simulink model "pam_demod"  (R2024a)
settings: Solver=VariableStepAuto  StartTime=0.0  StopTime=10.0  RelTol=1e-3
libraries: dspfdesign x2, spsSampleandHoldLib x1

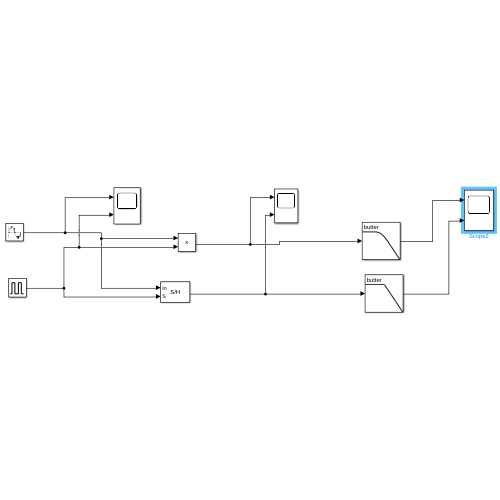
[thumbnail: Simulink's stored preview of the top-level diagram]
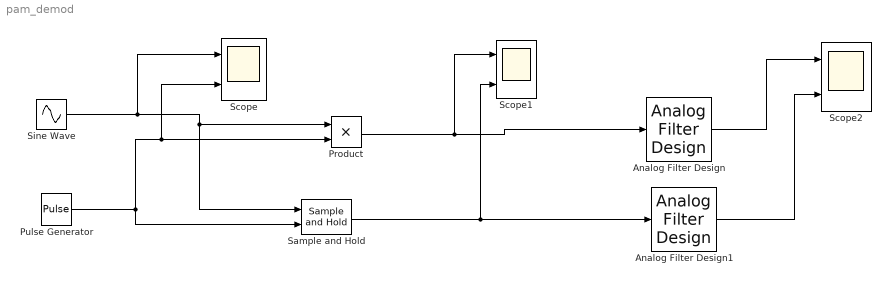
== system pam_demod ==
  Analog Filter Design : dspfdesign/Analog Filter Design  method=Butterworth  filttype=Lowpass  N=2  Wlo=1  Whi=80  Rp=2  Rs=40
  Analog Filter Design1 : dspfdesign/Analog Filter Design  method=Butterworth  filttype=Lowpass  N=8  Wlo=1.5  Whi=80  Rp=2  Rs=40
  Product : Product
  Pulse Generator : DiscretePulseGenerator  PulseType=Time based  Period=0.02  PulseWidth=50
  Sample and Hold : spsSampleandHoldLib/Sample and Hold  ic=0  Ts=0.001
      settings: LibrarySourceBlock=|
      | sps_lib/Control/Sample and
      | Hold
  Scope : Scope  NumInputPorts=2
  Scope1 : Scope  NumInputPorts=2
  Scope2 : Scope  NumInputPorts=2
  Sine Wave : Sin  Frequency=1.5  SampleTime=0.001
  wires:
  Analog Filter Design/1 -> Scope2/1
  Analog Filter Design1/1 -> Scope2/2
  Sample and Hold/1 -> Scope1/2, Analog Filter Design1/1
  Product/1 -> Scope1/1, Analog Filter Design/1
  Sine Wave/1 -> Scope/1, Sample and Hold/1, Product/1
  Pulse Generator/1 -> Sample and Hold/2, Scope/2, Product/2
